simulink model "test_nncACCsystem"  (R2019a)
settings: Solver=FixedStepAuto  StartTime=0.0  StopTime=T  RelTol=1e-3
values from neighbouring files (symbols this model uses):
  seed = randi([1001,2000])    [controller_comparison.m]
  t_gap = 1.4    [controller_comparison.m]
  Ts = 0.1    [controller_comparison.m]
  v0_ego = 20    [controller_comparison.m]
  v0_lead = 25    [controller_comparison.m]
  v_set = 30    [controller_comparison.m]
  x0_ego = 10    [controller_comparison.m]
  x0_lead = 50    [controller_comparison.m]
libraries: neural x35
(part 2 of 2)

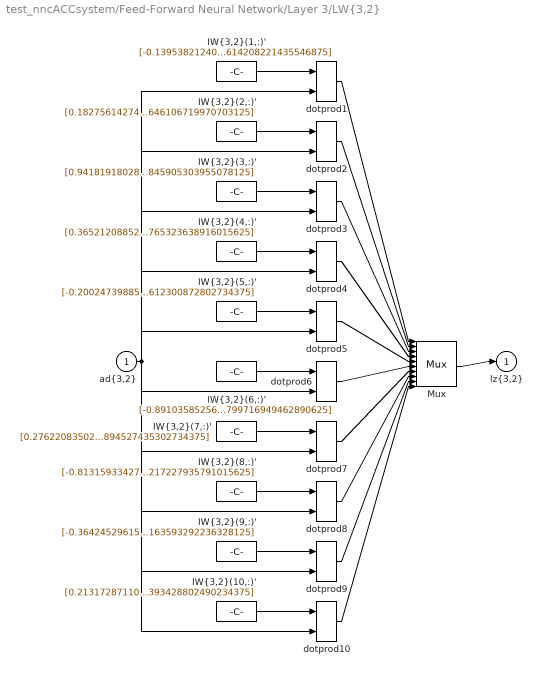
== system test_nncACCsystem/Feed-Forward Neural Network/Layer 3/LW{3,2} ==
  "ad{3,2}" : Inport  PortDimensions=10
      mask Display: e = 0.06;c1 = [120 230 180]/255;c2 = ([120 230 180]+0)/(256+128);c3 = ([120 230 180]+128)/(256+128);patch([0 1 1 0],[0 0 1 1],c1);patch([0 1 1 1-e 1-e 0+e],[0 0 1 1-e 0+e 0+e],c2);patch([0 0 1 1-e 0+e 0+e],[0 1 1 1-e 1-e 0+e],c3);plot([0 1 1 0 0],[0 0 1 1 0]);
  "IW{3,2}(1,:)'" : Constant  Value=[-0.139538212407251283053710722015239298343658447265625;-0.19790003605762507277177064679563045501708984375;-0.959037115574295828679396436200477182865142822265625;0.5612193739743556175625371906789951026439666748046875;-0.5779478947887424222784602534375153481960296630859375;-0.7662561031965660074405377599759958684444427490234375;-0.98475836290268592421170978923328220844268798828125;-0.5053012825411549169274394444073550403118133544921875;-0.9336308382616766987638357022660784423351287841796875;-0.2080982142762177744543805602006614208221435546875]
      mask Display: e = 0.06;c1 = [120 150 230]/255;c2 = ([120 150 230]+0)/383;c3 = ([120 150 230]+128)/383;patch([0 1 1 0],[0 0 1 1],c1);patch([0 1 1 1-e 1-e 0+e],[0 0 1 1-e 0+e 0+e],c2);patch([0 0 1 1-e 0+e 0+e],[0 1 1 1-e 1-e 0+e],c3);plot([0 1 1 0 0],[0 0 1 1 0]);disp('weights');
  "IW{3,2}(10,:)'" : Constant  Value=[0.2131728711042859547575289980159141123294830322265625;0.53527697480875335855898811132647097110748291015625;0.57061434804256705444203134902636520564556121826171875;-0.163801537499838445466338043843279592692852020263671875;-0.45460606753174948035933766732341609895229339599609375;-0.87898338986927881943955753740738146007061004638671875;-0.249828799907973853056120105975423939526081085205078125;0.1019888815948213067752448068858939222991466522216796875;0.79043697700747295176171292041544802486896514892578125;-0.654855157351684535882441196008585393428802490234375]
      mask Display: e = 0.06;c1 = [120 150 230]/255;c2 = ([120 150 230]+0)/383;c3 = ([120 150 230]+128)/383;patch([0 1 1 0],[0 0 1 1],c1);patch([0 1 1 1-e 1-e 0+e],[0 0 1 1-e 0+e 0+e],c2);patch([0 0 1 1-e 0+e 0+e],[0 1 1 1-e 1-e 0+e],c3);plot([0 1 1 0 0],[0 0 1 1 0]);disp('weights');
  "IW{3,2}(2,:)'" : Constant  Value=[0.1827561427442849772972977007157169282436370849609375;0.959150581481346353740491395001299679279327392578125;-0.82244446351649969084718350131879560649394989013671875;-0.2598968397235574823156412094249390065670013427734375;0.63276739210867283258465931794489733874797821044921875;0.033099615736605247917623273679055273532867431640625;-0.58074664297428935100242597400210797786712646484375;-0.7322195652337886162541735757258720695972442626953125;0.29804948258563579432944834479712881147861480712890625;-0.2475352156054970720333585632033646106719970703125]
      mask Display: e = 0.06;c1 = [120 150 230]/255;c2 = ([120 150 230]+0)/383;c3 = ([120 150 230]+128)/383;patch([0 1 1 0],[0 0 1 1],c1);patch([0 1 1 1-e 1-e 0+e],[0 0 1 1-e 0+e 0+e],c2);patch([0 0 1 1-e 0+e 0+e],[0 1 1 1-e 1-e 0+e],c3);plot([0 1 1 0 0],[0 0 1 1 0]);disp('weights');
  "IW{3,2}(3,:)'" : Constant  Value=[0.94181918028186561997472381335683166980743408203125;0.57300312098588446207969582246732898056507110595703125;-0.450026233254333940525526713827275671064853668212890625;0.07744227772075305826771085548898554407060146331787109375;-0.40354263366091325249129795338376425206661224365234375;0.69750454949859641562426304517430253326892852783203125;0.492389965757495884357552995425066910684108734130859375;0.66650256127062601496646720988792367279529571533203125;0.77117189705588795600732510138186626136302947998046875;-0.8880628980985125764391341363079845905303955078125]
      mask Display: e = 0.06;c1 = [120 150 230]/255;c2 = ([120 150 230]+0)/383;c3 = ([120 150 230]+128)/383;patch([0 1 1 0],[0 0 1 1],c1);patch([0 1 1 1-e 1-e 0+e],[0 0 1 1-e 0+e 0+e],c2);patch([0 0 1 1-e 0+e 0+e],[0 1 1 1-e 1-e 0+e],c3);plot([0 1 1 0 0],[0 0 1 1 0]);disp('weights');
  "IW{3,2}(4,:)'" : Constant  Value=[0.3652120885292491347939858314930461347103118896484375;0.10538838278812238946624546542807365767657756805419921875;0.5794369705555266758523202952346764504909515380859375;0.97384191438074985125439297917182557284832000732421875;-0.22407096442472151931468715702067129313945770263671875;0.93940777160124688816011939707095734775066375732421875;0.600665336788242854026975692249834537506103515625;-0.038354363167429177117195848722985829226672649383544921875;0.382447394018453235009502577668172307312488555908203125;-0.7438945505216365550182899823994375765323638916015625]
      mask Display: e = 0.06;c1 = [120 150 230]/255;c2 = ([120 150 230]+0)/383;c3 = ([120 150 230]+128)/383;patch([0 1 1 0],[0 0 1 1],c1);patch([0 1 1 1-e 1-e 0+e],[0 0 1 1-e 0+e 0+e],c2);patch([0 0 1 1-e 0+e 0+e],[0 1 1 1-e 1-e 0+e],c3);plot([0 1 1 0 0],[0 0 1 1 0]);disp('weights');
  "IW{3,2}(5,:)'" : Constant  Value=[-0.200247398850324831443003859021700918674468994140625;0.9246540322354508401048178711789660155773162841796875;0.0631463603622393065961659885942935943603515625;-0.720141487177964112476047375821508467197418212890625;-0.9604687807218745820847516370122320950031280517578125;0.4630495998965857840090620811679400503635406494140625;-0.3163042207864179555798500587115995585918426513671875;-0.3184061776728033255068339713034220039844512939453125;-0.491151390728998382684267198783345520496368408203125;-0.796041395844861110475676468922756612300872802734375]
      mask Display: e = 0.06;c1 = [120 150 230]/255;c2 = ([120 150 230]+0)/383;c3 = ([120 150 230]+128)/383;patch([0 1 1 0],[0 0 1 1],c1);patch([0 1 1 1-e 1-e 0+e],[0 0 1 1-e 0+e 0+e],c2);patch([0 0 1 1-e 0+e 0+e],[0 1 1 1-e 1-e 0+e],c3);plot([0 1 1 0 0],[0 0 1 1 0]);disp('weights');
  "IW{3,2}(6,:)'" : Constant  Value=[-0.891035852569122877042673280811868607997894287109375;-1.08643434791817039553052381961606442928314208984375;0.87655291290389047986764126108027994632720947265625;0.36780396557821337655269644528743810951709747314453125;0.1790524870930310930017270720782107673585414886474609375;0.0235584874563358574739435624678662861697375774383544921875;-0.9000325791739312020212082643411122262477874755859375;-0.4019175043789033896501905473996885120868682861328125;-0.15036225410887638087586992696742527186870574951171875;0.5127394290154720923879949623369611799716949462890625]
      mask Display: e = 0.06;c1 = [120 150 230]/255;c2 = ([120 150 230]+0)/383;c3 = ([120 150 230]+128)/383;patch([0 1 1 0],[0 0 1 1],c1);patch([0 1 1 1-e 1-e 0+e],[0 0 1 1-e 0+e 0+e],c2);patch([0 0 1 1-e 0+e 0+e],[0 1 1 1-e 1-e 0+e],c3);plot([0 1 1 0 0],[0 0 1 1 0]);disp('weights');
  "IW{3,2}(7,:)'" : Constant  Value=[0.27622083502342764660397733678109943866729736328125;-0.67312529827441525132059041425236500799655914306640625;-0.912982649264602930117007417720742523670196533203125;-0.0633341766820294249651368545528384856879711151123046875;0.089746838496134906382195595142547972500324249267578125;0.99108889282254020169915520455106161534786224365234375;-0.61415798000877963591648267538403160870075225830078125;0.42652353662872055650723268627189099788665771484375;0.5731258083229138211578401751467026770114898681640625;0.7320317203913953019167593083693645894527435302734375]
      mask Display: e = 0.06;c1 = [120 150 230]/255;c2 = ([120 150 230]+0)/383;c3 = ([120 150 230]+128)/383;patch([0 1 1 0],[0 0 1 1],c1);patch([0 1 1 1-e 1-e 0+e],[0 0 1 1-e 0+e 0+e],c2);patch([0 0 1 1-e 0+e 0+e],[0 1 1 1-e 1-e 0+e],c3);plot([0 1 1 0 0],[0 0 1 1 0]);disp('weights');
  "IW{3,2}(8,:)'" : Constant  Value=[-0.813159334274907497075446372036822140216827392578125;-0.996720431958193930910283597768284380435943603515625;0.6419857909532902251470432020141743123531341552734375;-0.45678540658129218599015075596980750560760498046875;-0.9627223870948053985330261639319360256195068359375;-0.308156951257052558190707713947631418704986572265625;0.1676679026504295233479524540598504245281219482421875;-0.21973240933396187557491430197842419147491455078125;-0.7256815974691595005907629456487484276294708251953125;0.9931896482608293386107334299595095217227935791015625]
      mask Display: e = 0.06;c1 = [120 150 230]/255;c2 = ([120 150 230]+0)/383;c3 = ([120 150 230]+128)/383;patch([0 1 1 0],[0 0 1 1],c1);patch([0 1 1 1-e 1-e 0+e],[0 0 1 1-e 0+e 0+e],c2);patch([0 0 1 1-e 0+e 0+e],[0 1 1 1-e 1-e 0+e],c3);plot([0 1 1 0 0],[0 0 1 1 0]);disp('weights');
  "IW{3,2}(9,:)'" : Constant  Value=[-0.3642452961578630521444210899062454700469970703125;0.51176596837130017281225491387885995209217071533203125;0.285960341372419935002113788868882693350315093994140625;0.363432631060336575057334584926138631999492645263671875;-0.2326807092637211693553211944163194857537746429443359375;-0.321421314042224681717385692536481656134128570556640625;0.82398746726408644835970562780858017504215240478515625;-0.419655047359981214771806889984873123466968536376953125;0.63079976641760426847582721165963448584079742431640625;-0.803043862694039933813883180846460163593292236328125]
      mask Display: e = 0.06;c1 = [120 150 230]/255;c2 = ([120 150 230]+0)/383;c3 = ([120 150 230]+128)/383;patch([0 1 1 0],[0 0 1 1],c1);patch([0 1 1 1-e 1-e 0+e],[0 0 1 1-e 0+e 0+e],c2);patch([0 0 1 1-e 0+e 0+e],[0 1 1 1-e 1-e 0+e],c3);plot([0 1 1 0 0],[0 0 1 1 0]);disp('weights');
  Mux : Mux  Inputs=10
      mask Display: e = 0.06;c1 = [120 150 230]/255;c2 = ([120 150 230]+0)/383;c3 = ([120 150 230]+128)/383;patch([0 1 1 0],[0 0 1 1],c1);patch([0 1 1 1-e 1-e 0+e],[0 0 1 1-e 0+e 0+e],c2);patch([0 0 1 1-e 0+e 0+e],[0 1 1 1-e 1-e 0+e],c3);plot([0 1 1 0 0],[0 0 1 1 0]);disp('Mux');
  dotprod{1..10} (10 alike) : neural/Weight Functions/dotprod
  "lz{3,2}" : Outport
      mask Display: e = 0.06;c1 = [120 230 180]/255;c2 = ([120 230 180]+0)/(256+128);c3 = ([120 230 180]+128)/(256+128);patch([0 1 1 0],[0 0 1 1],c1);patch([0 1 1 1-e 1-e 0+e],[0 0 1 1-e 0+e 0+e],c2);patch([0 0 1 1-e 0+e 0+e],[0 1 1 1-e 1-e 0+e],c3);plot([0 1 1 0 0],[0 0 1 1 0]);
  wires:
  "IW{3,2}(1,:)'"/1 -> dotprod1/1
  "ad{3,2}"/1 -> dotprod1/2, dotprod2/2, dotprod3/2, dotprod4/2, dotprod5/2, dotprod6/2, dotprod7/2, dotprod8/2, dotprod9/2, dotprod10/2
  dotprod1/1 -> Mux/1
  "IW{3,2}(2,:)'"/1 -> dotprod2/1
  dotprod2/1 -> Mux/2
  "IW{3,2}(3,:)'"/1 -> dotprod3/1
  dotprod3/1 -> Mux/3
  "IW{3,2}(4,:)'"/1 -> dotprod4/1
  dotprod4/1 -> Mux/4
  "IW{3,2}(5,:)'"/1 -> dotprod5/1
  dotprod5/1 -> Mux/5
  "IW{3,2}(6,:)'"/1 -> dotprod6/1
  dotprod6/1 -> Mux/6
  "IW{3,2}(7,:)'"/1 -> dotprod7/1
  dotprod7/1 -> Mux/7
  "IW{3,2}(8,:)'"/1 -> dotprod8/1
  dotprod8/1 -> Mux/8
  "IW{3,2}(9,:)'"/1 -> dotprod9/1
  dotprod9/1 -> Mux/9
  "IW{3,2}(10,:)'"/1 -> dotprod10/1
  dotprod10/1 -> Mux/10
  Mux/1 -> "lz{3,2}"/1

== system test_nncACCsystem/Feed-Forward Neural Network/Layer 4/Delays 1 ==
  "p{4}" : Inport  PortDimensions=10
      mask Display: e = 0.06;c1 = [120 230 180]/255;c2 = ([120 230 180]+0)/(256+128);c3 = ([120 230 180]+128)/(256+128);patch([0 1 1 0],[0 0 1 1],c1);patch([0 1 1 1-e 1-e 0+e],[0 0 1 1-e 0+e 0+e],c2);patch([0 0 1 1-e 0+e 0+e],[0 1 1 1-e 1-e 0+e],c3);plot([0 1 1 0 0],[0 0 1 1 0]);
  mux : Mux  Inputs=1
      mask Display: e = 0.06;c1 = [120 150 230]/255;c2 = ([120 150 230]+0)/383;c3 = ([120 150 230]+128)/383;patch([0 1 1 0],[0 0 1 1],c1);patch([0 1 1 1-e 1-e 0+e],[0 0 1 1-e 0+e 0+e],c2);patch([0 0 1 1-e 0+e 0+e],[0 1 1 1-e 1-e 0+e],c3);plot([0 1 1 0 0],[0 0 1 1 0]);disp('Mux')
  "pd{4,3}" : Outport
      mask Display: e = 0.06;c1 = [120 230 180]/255;c2 = ([120 230 180]+0)/(256+128);c3 = ([120 230 180]+128)/(256+128);patch([0 1 1 0],[0 0 1 1],c1);patch([0 1 1 1-e 1-e 0+e],[0 0 1 1-e 0+e 0+e],c2);patch([0 0 1 1-e 0+e 0+e],[0 1 1 1-e 1-e 0+e],c3);plot([0 1 1 0 0],[0 0 1 1 0]);
  wires:
  "p{4}"/1 -> mux/1
  mux/1 -> "pd{4,3}"/1

== system test_nncACCsystem/Feed-Forward Neural Network/Layer 4/LW{4,3} ==
  "ad{4,3}" : Inport  PortDimensions=10
      mask Display: e = 0.06;c1 = [120 230 180]/255;c2 = ([120 230 180]+0)/(256+128);c3 = ([120 230 180]+128)/(256+128);patch([0 1 1 0],[0 0 1 1],c1);patch([0 1 1 1-e 1-e 0+e],[0 0 1 1-e 0+e 0+e],c2);patch([0 0 1 1-e 0+e 0+e],[0 1 1 1-e 1-e 0+e],c3);plot([0 1 1 0 0],[0 0 1 1 0]);
  "IW{4,3}(1,:)'" : Constant  Value=[0.1408732832090129338808992542908526957035064697265625;-1.5889203220824726849220998037282015502569265663623809814453125e-05;0.539111600731424278620806944672949612140655517578125;-0.392902322309608142969494792851037345826625823974609375;-0.252675767184797894771008941461332142353057861328125;0.5041687608851865842751749369199387729167938232421875;-0.253424070270702461726841647760011255741119384765625;0.2378633444540791952448444135370664298534393310546875;0.274989415612188980997387943716603331267833709716796875;-0.313494451687272857043353724293410778045654296875]
      mask Display: e = 0.06;c1 = [120 150 230]/255;c2 = ([120 150 230]+0)/383;c3 = ([120 150 230]+128)/383;patch([0 1 1 0],[0 0 1 1],c1);patch([0 1 1 1-e 1-e 0+e],[0 0 1 1-e 0+e 0+e],c2);patch([0 0 1 1-e 0+e 0+e],[0 1 1 1-e 1-e 0+e],c3);plot([0 1 1 0 0],[0 0 1 1 0]);disp('weights');
  Mux : Mux  Inputs=1
      mask Display: e = 0.06;c1 = [120 150 230]/255;c2 = ([120 150 230]+0)/383;c3 = ([120 150 230]+128)/383;patch([0 1 1 0],[0 0 1 1],c1);patch([0 1 1 1-e 1-e 0+e],[0 0 1 1-e 0+e 0+e],c2);patch([0 0 1 1-e 0+e 0+e],[0 1 1 1-e 1-e 0+e],c3);plot([0 1 1 0 0],[0 0 1 1 0]);disp('Mux');
  dotprod1 : neural/Weight Functions/dotprod
  "lz{4,3}" : Outport
      mask Display: e = 0.06;c1 = [120 230 180]/255;c2 = ([120 230 180]+0)/(256+128);c3 = ([120 230 180]+128)/(256+128);patch([0 1 1 0],[0 0 1 1],c1);patch([0 1 1 1-e 1-e 0+e],[0 0 1 1-e 0+e 0+e],c2);patch([0 0 1 1-e 0+e 0+e],[0 1 1 1-e 1-e 0+e],c3);plot([0 1 1 0 0],[0 0 1 1 0]);
  wires:
  "IW{4,3}(1,:)'"/1 -> dotprod1/1
  "ad{4,3}"/1 -> dotprod1/2
  dotprod1/1 -> Mux/1
  Mux/1 -> "lz{4,3}"/1
